simulink model "ChemicalVersusElectricSynapse"  (Simulink 7.1)
settings: Solver=ode45  StartTime=0.0  StopTime=1  RelTol=1e-3
libraries: NeuroModelerLibrary x5
settings Model: Creator=Tim  LastModifiedBy=Timba

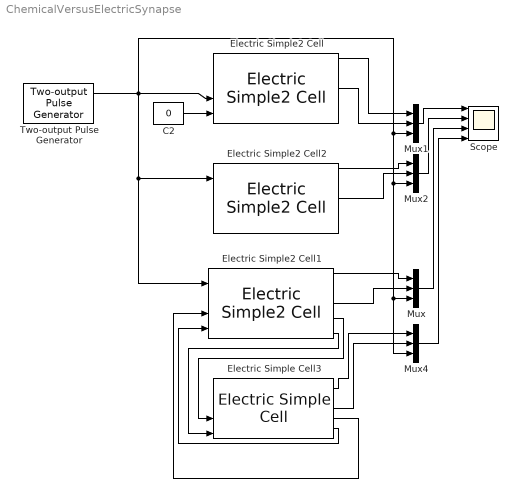
== system ChemicalVersusElectricSynapse ==
  C2 : Constant  Value=0  OutDataType=sfix(16)  OutScaling=2^0
  Electric Simple Cell3 : NeuroModelerLibrary/Simple Cells/Electric Simple Cell  SystemSampleTime=-1
  Electric Simple2 Cell : NeuroModelerLibrary/Simple Cells/Electric Simple2 Cell  SystemSampleTime=-1
  Electric Simple2 Cell1 : NeuroModelerLibrary/Simple Cells/Electric Simple2 Cell  SystemSampleTime=-1
  Electric Simple2 Cell2 : NeuroModelerLibrary/Simple Cells/Electric Simple2 Cell  SystemSampleTime=-1
  Mux{,1..2,4} (4 alike) : Mux  Inputs=3
  Scope : Scope  NumInputPorts=4
      settings: TimeRange=1  YMin=-0.021~-0.021~-0.021~-0.021  YMax=0.011~0.011~0.011~0.011  MaxDataPoints=50000
  Two-output Pulse Generator : NeuroModelerLibrary/Support/Two-output Pulse Generator  SystemSampleTime=-1  A=1  P1=200  P2=200  PW=1  ST=0.001  OOn1=0.2  OOff1=0.8  OOn2=0.2  OOff2=0.8
  wires:
  C2/1 -> Electric Simple2 Cell/4
  Two-output Pulse Generator/1 -> Electric Simple2 Cell/3, Mux1/3, Mux/3, Mux4/3, Mux2/3, Electric Simple2 Cell1/1, Electric Simple2 Cell2/1
  Mux/1 -> Scope/3
  Electric Simple2 Cell/3 -> Mux1/2
  Electric Simple2 Cell1/3 -> Mux/2
  Electric Simple Cell3/3 -> Mux4/2
  Electric Simple2 Cell1/4 -> Electric Simple Cell3/3
  Electric Simple2 Cell1/5 -> Electric Simple Cell3/4
  Electric Simple2 Cell/1 -> Mux1/1
  Mux1/1 -> Scope/1
  Electric Simple Cell3/1 -> Mux4/1
  Mux4/1 -> Scope/4
  Electric Simple2 Cell1/1 -> Mux/1
  Electric Simple2 Cell2/1 -> Mux2/1
  Electric Simple2 Cell2/3 -> Mux2/2
  Mux2/1 -> Scope/2
  Electric Simple Cell3/4 -> Electric Simple2 Cell1/3
  Electric Simple Cell3/5 -> Electric Simple2 Cell1/4
